simulink model "foc5"  (R2018a)
settings: Solver=ode45  StartTime=0.0  StopTime=0.5  MaxStep=2.0E-6  RelTol=1e-3
libraries: simulink x6, powerlib x4, powerlib_meascontrol x2
settings Model: Creator=R-YDL  LastModifiedBy=R-YDL

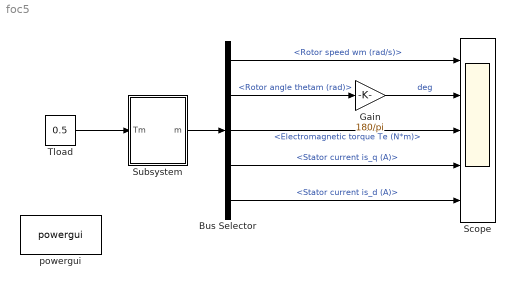
== system foc5 ==
  Bus Selector : BusSelector  OutputSignals=Rotor speed wm (rad/s),Rotor angle thetam (rad),Electromagnetic torque Te (N*m),Stator current is_q (A),Stator current is_d (A)
  Gain : Gain  Gain=180/pi
  Scope : Scope  NumInputPorts=5
  Subsystem : Subsystem  mask{Va=0, Vb=0, Vc=0, t0=0}
  Tload : Constant  Value=0.5
  powergui : powerlib/powergui  Priority=1  SimulationMode=Discrete  SampleTime=2e-6  frequency=60  Iterations=50  frequencyindice=0  Pbase=100e6  ErrMax=1e-4  UnitsV=kV  UnitsW=MW  buscounter=0  FunctionMessages=off  echomessages=off  EnableUseOfTLC=off  CurrentSourceSwitches=off  DisableSnubberDevices=off  DisableRonSwitches=off  DisableVfSwitches=off  DisplayEquations=off  SolverType=Tustin/Backward Euler (TBE)  Interpol=off  ExternalGateDelay=off  methode=off  Ts=100  x0status=blocks  SPID=on  SwTol=0  HookPort=off  RestoreLinks=warning  ResistiveCurrentMeasurement=off  Frange=[0:2:500]  Ylog=off  Xlog=on  ShowGrid=off  save=off  variable=ZData  structure=0  ZoomFFT=off  StartTime=0.0  cycles=1  DisplayStyle=1  fundamental=60  FreqAxis=off  MaxFrequency=1000  frequencyindicesteady=1  RmsSteady=1  display=off
  wires:
  Bus Selector/5 -> Scope/5  "<Stator current is_d (A)>"
  Bus Selector/4 -> Scope/4  "<Stator current is_q (A)>"
  Subsystem/1(m) -> Bus Selector/1
  Bus Selector/2 -> Gain/1  "<Rotor angle thetam (rad)>"
  Bus Selector/3 -> Scope/3  "<Electromagnetic torque Te (N*m)>"
  Gain/1 -> Scope/2  "deg"
  Bus Selector/1 -> Scope/1  "<Rotor speed wm (rad/s)>"
  Tload/1 -> Subsystem/1(Tm)

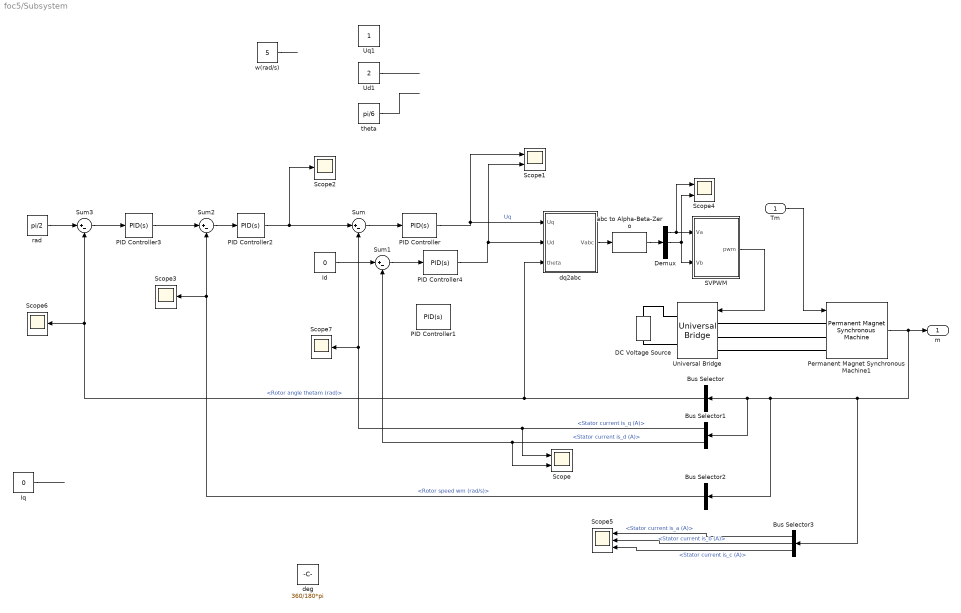
== system foc5/Subsystem ==
  Tm : Inport
  Bus Selector : BusSelector  OutputSignals=Rotor angle thetam (rad)
  Bus Selector1 : BusSelector  OutputSignals=Stator current is_q (A),Stator current is_d (A)
  Bus Selector2 : BusSelector  OutputSignals=Rotor speed wm (rad/s)
  Bus Selector3 : BusSelector  OutputSignals=Stator current is_a (A),Stator current is_b (A),Stator current is_c (A)
  DC Voltage Source : powerlib/Electrical Sources/DC Voltage Source  Amplitude=100  Measurements=None
  Demux : Demux  Outputs=3
  Id : Constant  Value=0
  Iq : Constant  Value=0
  PID Controller : simulink/Continuous/PID Controller  Controller=PID  TimeDomain=Continuous-time  SampleTime=-1  IntegratorMethod=Forward Euler  FilterMethod=Forward Euler  Form=Parallel  UseFilter=on  ControllerParametersSource=internal  P=50  I=5000  D=0  N=100  InitialConditionSource=internal  InitialConditionForIntegrator=0  InitialConditionForFilter=0  ExternalReset=none  LimitOutput=on  UpperSaturationLimit=100  LowerSaturationLimit=-100  LinearizeAsGain=on  AntiWindupMode=none  Kb=1  TrackingMode=off  Kt=1  PParamMin=[]  PParamMax=[]  IParamMin=[]  IParamMax=[]  DParamMin=[]  DParamMax=[]  NParamMin=[]  NParamMax=[]  KbParamMin=[]  KbParamMax=[]  KtParamMin=[]  KtParamMax=[]  POutMin=[]  POutMax=[]  IOutMin=[]  IOutMax=[]  DOutMin=[]  DOutMax=[]  NOutMin=[]  NOutMax=[]  KbOutMin=[]  KbOutMax=[]  KtOutMin=[]  KtOutMax=[]  IntegratorOutMin=[]  IntegratorOutMax=[]  FilterOutMin=[]  FilterOutMax=[]  SumOutMin=[]  SumOutMax=[]  SumI1OutMin=[]  SumI1OutMax=[]  SumI2OutMin=[]  SumI2OutMax=[]  SumI3OutMin=[]  SumI3OutMax=[]  SumDOutMin=[]  SumDOutMax=[]  SaturationOutMin=[]  SaturationOutMax=[]  IntegratorContinuousStateAttributes=''  IntegratorStateMustResolveToSignalObject=off  IntegratorRTWStateStorageClass=Auto  FilterContinuousStateAttributes=''  FilterStateMustResolveToSignalObject=off  FilterRTWStateStorageClass=Auto  DifferentiatorICPrevScaledInput=0  DifferentiatorOutMin=[]  DifferentiatorOutMax=[]  FilterDiffOutCoefMin=[]  FilterDiffOutCoefMax=[]  SumDenOutMin=[]  SumDenOutMax=[]  SumNumOutMin=[]  SumNumOutMax=[]  ReciprocalOutMin=[]  ReciprocalOutMax=[]  DivideOutMin=[]  DivideOutMax=[]  TunerSelectOption=Transfer Function Based (PID Tuner App)
  PID Controller1 : simulink/Continuous/PID Controller  Controller=PID  TimeDomain=Continuous-time  SampleTime=-1  IntegratorMethod=Forward Euler  FilterMethod=Forward Euler  Form=Parallel  UseFilter=on  ControllerParametersSource=internal  P=50  I=5000  D=0  N=100  InitialConditionSource=internal  InitialConditionForIntegrator=0  InitialConditionForFilter=0  ExternalReset=none  LimitOutput=on  UpperSaturationLimit=100  LowerSaturationLimit=-100  LinearizeAsGain=on  AntiWindupMode=none  Kb=1  TrackingMode=off  Kt=1  PParamMin=[]  PParamMax=[]  IParamMin=[]  IParamMax=[]  DParamMin=[]  DParamMax=[]  NParamMin=[]  NParamMax=[]  KbParamMin=[]  KbParamMax=[]  KtParamMin=[]  KtParamMax=[]  POutMin=[]  POutMax=[]  IOutMin=[]  IOutMax=[]  DOutMin=[]  DOutMax=[]  NOutMin=[]  NOutMax=[]  KbOutMin=[]  KbOutMax=[]  KtOutMin=[]  KtOutMax=[]  IntegratorOutMin=[]  IntegratorOutMax=[]  FilterOutMin=[]  FilterOutMax=[]  SumOutMin=[]  SumOutMax=[]  SumI1OutMin=[]  SumI1OutMax=[]  SumI2OutMin=[]  SumI2OutMax=[]  SumI3OutMin=[]  SumI3OutMax=[]  SumDOutMin=[]  SumDOutMax=[]  SaturationOutMin=[]  SaturationOutMax=[]  IntegratorContinuousStateAttributes=''  IntegratorStateMustResolveToSignalObject=off  IntegratorRTWStateStorageClass=Auto  FilterContinuousStateAttributes=''  FilterStateMustResolveToSignalObject=off  FilterRTWStateStorageClass=Auto  DifferentiatorICPrevScaledInput=0  DifferentiatorOutMin=[]  DifferentiatorOutMax=[]  FilterDiffOutCoefMin=[]  FilterDiffOutCoefMax=[]  SumDenOutMin=[]  SumDenOutMax=[]  SumNumOutMin=[]  SumNumOutMax=[]  ReciprocalOutMin=[]  ReciprocalOutMax=[]  DivideOutMin=[]  DivideOutMax=[]  TunerSelectOption=Transfer Function Based (PID Tuner App)
  PID Controller2 : simulink/Continuous/PID Controller  Controller=PID  TimeDomain=Continuous-time  SampleTime=-1  IntegratorMethod=Forward Euler  FilterMethod=Forward Euler  Form=Parallel  UseFilter=on  ControllerParametersSource=internal  P=20  I=500  D=0  N=100  InitialConditionSource=internal  InitialConditionForIntegrator=0  InitialConditionForFilter=0  ExternalReset=none  LimitOutput=on  UpperSaturationLimit=100  LowerSaturationLimit=-100  LinearizeAsGain=on  AntiWindupMode=none  Kb=1  TrackingMode=off  Kt=1  PParamMin=[]  PParamMax=[]  IParamMin=[]  IParamMax=[]  DParamMin=[]  DParamMax=[]  NParamMin=[]  NParamMax=[]  KbParamMin=[]  KbParamMax=[]  KtParamMin=[]  KtParamMax=[]  POutMin=[]  POutMax=[]  IOutMin=[]  IOutMax=[]  DOutMin=[]  DOutMax=[]  NOutMin=[]  NOutMax=[]  KbOutMin=[]  KbOutMax=[]  KtOutMin=[]  KtOutMax=[]  IntegratorOutMin=[]  IntegratorOutMax=[]  FilterOutMin=[]  FilterOutMax=[]  SumOutMin=[]  SumOutMax=[]  SumI1OutMin=[]  SumI1OutMax=[]  SumI2OutMin=[]  SumI2OutMax=[]  SumI3OutMin=[]  SumI3OutMax=[]  SumDOutMin=[]  SumDOutMax=[]  SaturationOutMin=[]  SaturationOutMax=[]  IntegratorContinuousStateAttributes=''  IntegratorStateMustResolveToSignalObject=off  IntegratorRTWStateStorageClass=Auto  FilterContinuousStateAttributes=''  FilterStateMustResolveToSignalObject=off  FilterRTWStateStorageClass=Auto  DifferentiatorICPrevScaledInput=0  DifferentiatorOutMin=[]  DifferentiatorOutMax=[]  FilterDiffOutCoefMin=[]  FilterDiffOutCoefMax=[]  SumDenOutMin=[]  SumDenOutMax=[]  SumNumOutMin=[]  SumNumOutMax=[]  ReciprocalOutMin=[]  ReciprocalOutMax=[]  DivideOutMin=[]  DivideOutMax=[]  TunerSelectOption=Transfer Function Based (PID Tuner App)
  PID Controller3 : simulink/Continuous/PID Controller  Controller=PID  TimeDomain=Continuous-time  SampleTime=-1  IntegratorMethod=Forward Euler  FilterMethod=Forward Euler  Form=Parallel  UseFilter=on  ControllerParametersSource=internal  P=3  I=0  D=0  N=100  InitialConditionSource=internal  InitialConditionForIntegrator=0  InitialConditionForFilter=0  ExternalReset=none  LimitOutput=on  UpperSaturationLimit=100  LowerSaturationLimit=-100  LinearizeAsGain=on  AntiWindupMode=none  Kb=1  TrackingMode=off  Kt=1  PParamMin=[]  PParamMax=[]  IParamMin=[]  IParamMax=[]  DParamMin=[]  DParamMax=[]  NParamMin=[]  NParamMax=[]  KbParamMin=[]  KbParamMax=[]  KtParamMin=[]  KtParamMax=[]  POutMin=[]  POutMax=[]  IOutMin=[]  IOutMax=[]  DOutMin=[]  DOutMax=[]  NOutMin=[]  NOutMax=[]  KbOutMin=[]  KbOutMax=[]  KtOutMin=[]  KtOutMax=[]  IntegratorOutMin=[]  IntegratorOutMax=[]  FilterOutMin=[]  FilterOutMax=[]  SumOutMin=[]  SumOutMax=[]  SumI1OutMin=[]  SumI1OutMax=[]  SumI2OutMin=[]  SumI2OutMax=[]  SumI3OutMin=[]  SumI3OutMax=[]  SumDOutMin=[]  SumDOutMax=[]  SaturationOutMin=[]  SaturationOutMax=[]  IntegratorContinuousStateAttributes=''  IntegratorStateMustResolveToSignalObject=off  IntegratorRTWStateStorageClass=Auto  FilterContinuousStateAttributes=''  FilterStateMustResolveToSignalObject=off  FilterRTWStateStorageClass=Auto  DifferentiatorICPrevScaledInput=0  DifferentiatorOutMin=[]  DifferentiatorOutMax=[]  FilterDiffOutCoefMin=[]  FilterDiffOutCoefMax=[]  SumDenOutMin=[]  SumDenOutMax=[]  SumNumOutMin=[]  SumNumOutMax=[]  ReciprocalOutMin=[]  ReciprocalOutMax=[]  DivideOutMin=[]  DivideOutMax=[]  TunerSelectOption=Transfer Function Based (PID Tuner App)
  PID Controller4 : simulink/Continuous/PID Controller  Controller=PID  TimeDomain=Continuous-time  SampleTime=-1  IntegratorMethod=Forward Euler  FilterMethod=Forward Euler  Form=Parallel  UseFilter=on  ControllerParametersSource=internal  P=50  I=5000  D=0  N=100  InitialConditionSource=internal  InitialConditionForIntegrator=0  InitialConditionForFilter=0  ExternalReset=none  LimitOutput=on  UpperSaturationLimit=100  LowerSaturationLimit=-100  LinearizeAsGain=on  AntiWindupMode=none  Kb=1  TrackingMode=off  Kt=1  PParamMin=[]  PParamMax=[]  IParamMin=[]  IParamMax=[]  DParamMin=[]  DParamMax=[]  NParamMin=[]  NParamMax=[]  KbParamMin=[]  KbParamMax=[]  KtParamMin=[]  KtParamMax=[]  POutMin=[]  POutMax=[]  IOutMin=[]  IOutMax=[]  DOutMin=[]  DOutMax=[]  NOutMin=[]  NOutMax=[]  KbOutMin=[]  KbOutMax=[]  KtOutMin=[]  KtOutMax=[]  IntegratorOutMin=[]  IntegratorOutMax=[]  FilterOutMin=[]  FilterOutMax=[]  SumOutMin=[]  SumOutMax=[]  SumI1OutMin=[]  SumI1OutMax=[]  SumI2OutMin=[]  SumI2OutMax=[]  SumI3OutMin=[]  SumI3OutMax=[]  SumDOutMin=[]  SumDOutMax=[]  SaturationOutMin=[]  SaturationOutMax=[]  IntegratorContinuousStateAttributes=''  IntegratorStateMustResolveToSignalObject=off  IntegratorRTWStateStorageClass=Auto  FilterContinuousStateAttributes=''  FilterStateMustResolveToSignalObject=off  FilterRTWStateStorageClass=Auto  DifferentiatorICPrevScaledInput=0  DifferentiatorOutMin=[]  DifferentiatorOutMax=[]  FilterDiffOutCoefMin=[]  FilterDiffOutCoefMax=[]  SumDenOutMin=[]  SumDenOutMax=[]  SumNumOutMin=[]  SumNumOutMax=[]  ReciprocalOutMin=[]  ReciprocalOutMax=[]  DivideOutMin=[]  DivideOutMax=[]  TunerSelectOption=Transfer Function Based (PID Tuner App)
  Permanent Magnet Synchronous Machine1 : powerlib/Machines/Permanent Magnet Synchronous Machine  NbPhases=3  FluxDistribution=Sinusoidal  RotorType=Round  MechanicalLoad=Torque Tm  PresetModel=No  ShowDetailedParameters=on  MeasurementBus=off  Resistance=7  Inductance=8.5e-3  dqInductances=[8.5e-3,8.5e-3]  La=0.000395  MachineConstant=Flux linkage established by magnets (V.s)  Flux=0.1194  VoltageCst=21.6568  TorqueCst=0.1791  Flat=120  Mechanical=[0.0027 0.0424924 1 0]  PolePairs=4  InitialConditions=[0,t0, 0,0]  InitialConditions5ph=[0 0 0 0 0 0]  TsPowergui=0  TsBlock=-1  RefAngle=Aligned with phase A axis (original Park)
      settings: SourceProductName=Simscape Power Systems
  SVPWM : Subsystem  mask{T=1e-4, Ts=2e-6, Td=2e-6, Vdc=12}
      mask prompts: T "载波周期T(s)"; Ts "采样周期Ts"; Td "死区时间Td"; Vdc "直流母线电压Vdc"
  Scope : Scope  NumInputPorts=2
  Scope1 : Scope  NumInputPorts=2
  Scope{2..3,6..7} (4 alike) : Scope
  Scope4 : Scope  NumInputPorts=2
  Scope5 : Scope  NumInputPorts=3
  Sum{,1..3} (4 alike) : Sum  Inputs=|+-
  Ud1 : Constant  Value=2
  Universal Bridge : powerlib/Power Electronics/Universal Bridge  Arms=3  SnubberResistance=1e5  SnubberCapacitance=inf  Device=IGBT / Diodes  Ron=1e-3  Lon=0  ForwardVoltages="[  0  0  ]"  ForwardVoltage=0  GTOparameters=[ 10e-6 , 20e-6 ]  IGBTparameters=[ 1e-6 , 2e-6 ]  Measurements=None  Measurements_2=None  converterType=Rectifier
  Uq1 : Constant
  abc to Alpha-Beta-Zero : powerlib_meascontrol/Transformations/abc to Alpha-Beta-Zero
      settings: SourceProductName=Simscape Power Systems
  deg : Constant  Value=360/180*pi
  dq2abc : Subsystem
  rad : Constant  Value=pi/2
  theta : Constant  Value=pi/6
  w(rad/s) : Constant  Value=5
  m : Outport
  wires:
  Tm/1 -> Permanent Magnet Synchronous Machine1/1
  Permanent Magnet Synchronous Machine1/1 -> m/1, Bus Selector3/1, Bus Selector2/1, Bus Selector1/1, Bus Selector/1
  Sum/1 -> PID Controller/1
  Id/1 -> Sum1/1
  PID Controller/1 -> dq2abc/1(Uq), Scope1/1  "Uq"
  Bus Selector1/1 -> Scope/1, Scope7/1, Sum/2  "<Stator current is_q (A)>"
  Bus Selector1/2 -> Scope/2, Sum1/2  "<Stator current is_d (A)>"
  PID Controller2/1 -> Sum/1, Scope2/1
  Sum2/1 -> PID Controller2/1
  Bus Selector2/1 -> Scope3/1, Sum2/2  "<Rotor speed wm (rad/s)>"
  SVPWM/1(pwm) -> Universal Bridge/1
  Demux/1 -> Scope4/1, SVPWM/1(Va)
  Demux/2 -> Scope4/2, SVPWM/2(Vb)
  dq2abc/1(Vabc) -> abc to Alpha-Beta-Zero/1
  abc to Alpha-Beta-Zero/1 -> Demux/1
  Bus Selector3/1 -> Scope5/1  "<Stator current is_a (A)>"
  Bus Selector3/2 -> Scope5/2  "<Stator current is_b (A)>"
  Bus Selector3/3 -> Scope5/3  "<Stator current is_c (A)>"
  Bus Selector/1 -> dq2abc/3(theta), Scope6/1, Sum3/2  "<Rotor angle thetam (rad)>"
  rad/1 -> Sum3/1
  Sum3/1 -> PID Controller3/1
  w(rad/s)/1 -> ?
  PID Controller3/1 -> Sum2/1
  theta/1 -> ?
  Ud1/1 -> ?
  PID Controller4/1 -> Scope1/2, dq2abc/2(Ud)
  Sum1/1 -> PID Controller4/1
  Iq/1 -> ?
  connections:
  Universal Bridge/LConn2 -- Permanent Magnet Synchronous Machine1/LConn2
  Universal Bridge/LConn1 -- Permanent Magnet Synchronous Machine1/LConn1
  Universal Bridge/LConn3 -- Permanent Magnet Synchronous Machine1/LConn3
  Universal Bridge/RConn1 -- DC Voltage Source/RConn1
  Universal Bridge/RConn2 -- DC Voltage Source/LConn1

== system foc5/Subsystem/SVPWM ==
  Va : Inport
  Vb : Inport  Port=2
  Constant : Constant  Value=2/3*Vdc
  Divide : Product  Inputs=*/
  Divide1 : Product  Inputs=*/
  PWM : Subsystem
  Scope1 : Scope
  Scope2 : Scope
  Sec : Subsystem
  Subsystem5 : Subsystem
  pwm : Outport
  wires:
  Subsystem5/1(m(a,b,c)) -> Scope1/1, PWM/1("m_(a,b,c) ")
  PWM/1(pwm) -> pwm/1
  Sec/1(sec) -> Subsystem5/1(sec), Scope2/1
  Va/1 -> Divide/1
  Divide/1 -> Subsystem5/2(Va), Sec/1(Va)
  Vb/1 -> Divide1/1
  Divide1/1 -> Sec/2(Vb), Subsystem5/3(Vb)
  Constant/1 -> Divide1/2, Divide/2

== system foc5/Subsystem/dq2abc ==
  Uq : Inport
  Ud : Inport  Port=2
  theta : Inport  Port=3
  Mux : Mux  Inputs=3
  Subsystem : Subsystem
  Subsystem1 : Subsystem
  Subsystem3 : Subsystem
  Vabc : Outport
  wires:
  theta/1 -> Subsystem/3(theta), Subsystem1/3(theta), Subsystem3/3(theta)
  Ud/1 -> Subsystem3/2(Ud), Subsystem1/2(Ud), Subsystem/2(Ud)
  Uq/1 -> Subsystem3/1(Uq), Subsystem1/1(Uq), Subsystem/1(Uq)
  Subsystem/1(V) -> Mux/1
  Subsystem1/1(V) -> Mux/2
  Subsystem3/1(V) -> Mux/3
  Mux/1 -> Vabc/1

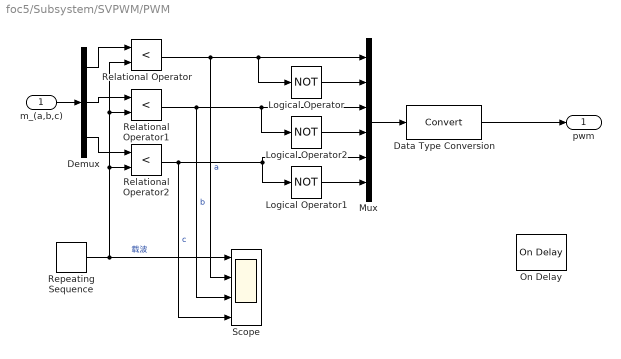
== system foc5/Subsystem/SVPWM/PWM ==
  "m_(a,b,c) " : Inport
  Data Type Conversion : DataTypeConversion
  Demux : Demux  Outputs=3
  Logical Operator : Logic  Operator=NOT  AllPortsSameDT=off  OutDataTypeStr=boolean
  Logical Operator1 : Logic  Operator=NOT  AllPortsSameDT=off  OutDataTypeStr=boolean
  Logical Operator2 : Logic  Operator=NOT  AllPortsSameDT=off  OutDataTypeStr=boolean
  Mux : Mux  Inputs=6
  On Delay : powerlib_meascontrol/Logic/On Delay  DelayType=On delay  delay=Td  ic=0  Ts=Ts
      settings: SourceProductName=Simscape Power Systems
  Relational Operator : RelationalOperator  Operator=<  OutDataTypeStr=boolean  RndMeth=Simplest
  Relational Operator1 : RelationalOperator  Operator=<  OutDataTypeStr=boolean  RndMeth=Simplest
  Relational Operator2 : RelationalOperator  Operator=<  OutDataTypeStr=boolean  RndMeth=Simplest
  Repeating Sequence : simulink/Sources/Repeating Sequence  rep_seq_t=[0 0.5 1]*T  rep_seq_y=[0 0.5 0]*T
  Scope : Scope  NumInputPorts=4
  pwm : Outport
  wires:
  Repeating Sequence/1 -> Relational Operator/2, Relational Operator1/2, Relational Operator2/2, Scope/1  "载波"
  Relational Operator/1 -> Mux/1, Logical Operator/1, Scope/2  "a"
  Relational Operator1/1 -> Logical Operator2/1, Mux/3, Scope/3  "b"
  Relational Operator2/1 -> Logical Operator1/1, Mux/5, Scope/4  "c"
  "m_(a,b,c) "/1 -> Demux/1
  Demux/1 -> Relational Operator/1
  Demux/2 -> Relational Operator1/1
  Demux/3 -> Relational Operator2/1
  Logical Operator/1 -> Mux/2
  Logical Operator2/1 -> Mux/4
  Logical Operator1/1 -> Mux/6
  Mux/1 -> Data Type Conversion/1
  Data Type Conversion/1 -> pwm/1

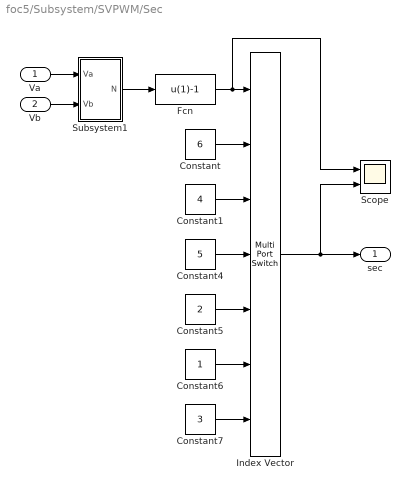
== system foc5/Subsystem/SVPWM/Sec ==
  Va : Inport
  Vb : Inport  Port=2
  Constant : Constant  Value=6
  Constant1 : Constant  Value=4
  Constant4 : Constant  Value=5
  Constant5 : Constant  Value=2
  Constant6 : Constant
  Constant7 : Constant  Value=3
  Fcn : Fcn  Expr=u(1)-1
  Index Vector : MultiPortSwitch  DataPortOrder=Zero-based contiguous  Inputs=6  zeroidx=on
  Scope : Scope  NumInputPorts=2
  Subsystem1 : Subsystem
  sec : Outport
  wires:
  Constant4/1 -> Index Vector/4
  Constant7/1 -> Index Vector/7
  Constant6/1 -> Index Vector/6
  Constant5/1 -> Index Vector/5
  Constant1/1 -> Index Vector/3
  Subsystem1/1("N ") -> Fcn/1
  Fcn/1 -> Scope/1, Index Vector/1
  Constant/1 -> Index Vector/2
  Va/1 -> Subsystem1/1(Va)
  Vb/1 -> Subsystem1/2("Vb ")
  Index Vector/1 -> sec/1, Scope/2

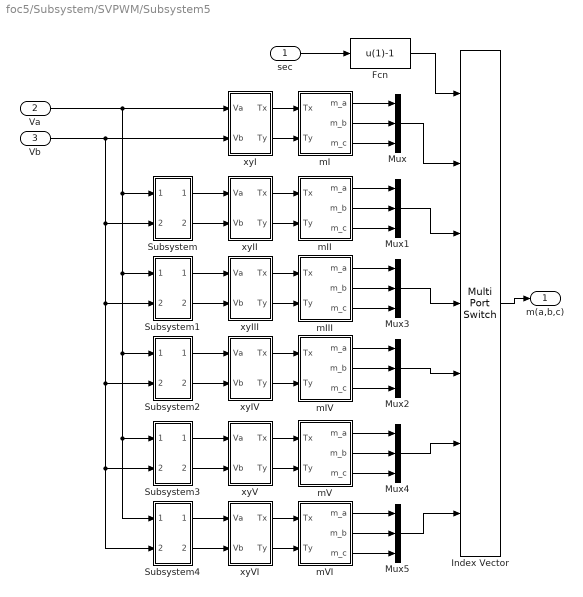
== system foc5/Subsystem/SVPWM/Subsystem5 ==
  sec : Inport
  Va : Inport  Port=2
  Vb : Inport  Port=3
  Fcn : Fcn  Expr=u(1)-1
  Index Vector : MultiPortSwitch  DataPortOrder=Zero-based contiguous  Inputs=6  zeroidx=on
  Mux{,1..5} (6 alike) : Mux  Inputs=3
  Subsystem : Subsystem
  Subsystem1 : Subsystem
  Subsystem2 : Subsystem
  Subsystem3 : Subsystem
  Subsystem4 : Subsystem
  mI : Subsystem
  mII : Subsystem
  mIII : Subsystem
  mIV : Subsystem
  mV : Subsystem
  mVI : Subsystem
  xyI : Subsystem
  xyII : Subsystem
  xyIII : Subsystem
  xyIV : Subsystem
  xyV : Subsystem
  xyVI : Subsystem
  m(a,b,c) : Outport
  wires:
  Subsystem2/1(Va') -> xyIV/1(Va)
  xyVI/2(Ty) -> mVI/2(Ty)
  mVI/1(m_a) -> Mux5/1
  Vb/1 -> Subsystem2/2(Vb), Subsystem4/2(Vb), Subsystem3/2(Vb), Subsystem1/2(Vb), Subsystem/2(Vb), xyI/2("Vb ")
  Subsystem2/2(Vb') -> xyIV/2("Vb ")
  mIV/3(m_c) -> Mux2/3
  Subsystem/1(Va') -> xyII/1(Va)
  Mux1/1 -> Index Vector/3
  Subsystem1/2(Vb') -> xyIII/2("Vb ")
  Va/1 -> Subsystem/1(Va), Subsystem4/1(Va), Subsystem3/1(Va), Subsystem2/1(Va), Subsystem1/1(Va), xyI/1(Va)
  mVI/2(m_b) -> Mux5/2
  Subsystem3/1(Va') -> xyV/1(Va)
  Mux/1 -> Index Vector/2
  xyIV/2(Ty) -> mIV/2(Ty)
  Mux4/1 -> Index Vector/6
  mVI/3(m_c) -> Mux5/3
  xyIV/1(Tx) -> mIV/1(Tx)
  xyI/1(Tx) -> mI/1("Tx ")
  mIV/2(m_b) -> Mux2/2
  Mux3/1 -> Index Vector/4
  xyI/2(Ty) -> mI/2("Ty ")
  Subsystem1/1(Va') -> xyIII/1(Va)
  mI/3(m_c) -> Mux/3
  xyIII/2(Ty) -> mIII/2(Ty)
  mI/2(m_b) -> Mux/2
  mI/1(m_a) -> Mux/1
  Subsystem4/1(Va') -> xyVI/1(Va)
  mIV/1(m_a) -> Mux2/1
  xyIII/1(Tx) -> mIII/1(Tx)
  xyII/2(Ty) -> mII/2("Ty ")
  xyII/1(Tx) -> mII/1("Tx ")
  Subsystem3/2(Vb') -> xyV/2("Vb ")
  Mux2/1 -> Index Vector/5
  Subsystem4/2(Vb') -> xyVI/2("Vb ")
  Mux5/1 -> Index Vector/7
  Subsystem/2(Vb') -> xyII/2("Vb ")
  xyVI/1(Tx) -> mVI/1(Tx)
  sec/1 -> Fcn/1
  Fcn/1 -> Index Vector/1
  mII/1(m_a) -> Mux1/1
  mII/2(m_b) -> Mux1/2
  mII/3(m_c) -> Mux1/3
  mIII/1(m_a) -> Mux3/1
  mIII/2(m_b) -> Mux3/2
  mIII/3(m_c) -> Mux3/3
  mV/1(m_a) -> Mux4/1
  mV/2(m_b) -> Mux4/2
  mV/3(m_c) -> Mux4/3
  Index Vector/1 -> m(a,b,c)/1
  xyV/1(Tx) -> mV/1(Tx)
  xyV/2(Ty) -> mV/2(Ty)

== system foc5/Subsystem/dq2abc/Subsystem ==
  Uq : Inport
  Ud : Inport  Port=2
  theta : Inport  Port=3
  Constant : Constant  Value=0
  Product : Product
  Product1 : Product
  Sum : Sum  Inputs=|-+
  Sum1 : Sum  Inputs=|++
  Trigonometric Function : Trigonometry
  Trigonometric Function1 : Trigonometry  Operator=cos
  V : Outport
  wires:
  Uq/1 -> Product/1
  Trigonometric Function1/1 -> Product1/2
  Trigonometric Function/1 -> Product/2
  Product1/1 -> Sum/2
  Product/1 -> Sum/1
  Sum/1 -> V/1
  Ud/1 -> Product1/1
  Sum1/1 -> Trigonometric Function/1, Trigonometric Function1/1
  theta/1 -> Sum1/1
  Constant/1 -> Sum1/2

== system foc5/Subsystem/dq2abc/Subsystem1 ==
  Uq : Inport
  Ud : Inport  Port=2
  theta : Inport  Port=3
  Constant : Constant  Value=-2*pi/3
  Product : Product
  Product1 : Product
  Sum : Sum  Inputs=|-+
  Sum1 : Sum  Inputs=|++
  Trigonometric Function : Trigonometry
  Trigonometric Function1 : Trigonometry  Operator=cos
  V : Outport
  wires:
  Uq/1 -> Product/1
  Trigonometric Function1/1 -> Product1/2
  Trigonometric Function/1 -> Product/2
  Product1/1 -> Sum/2
  Product/1 -> Sum/1
  Sum/1 -> V/1
  Ud/1 -> Product1/1
  Sum1/1 -> Trigonometric Function/1, Trigonometric Function1/1
  theta/1 -> Sum1/1
  Constant/1 -> Sum1/2

== system foc5/Subsystem/dq2abc/Subsystem3 ==
  Uq : Inport
  Ud : Inport  Port=2
  theta : Inport  Port=3
  Constant : Constant  Value=2*pi/3
  Product : Product
  Product1 : Product
  Sum : Sum  Inputs=|-+
  Sum1 : Sum  Inputs=|++
  Trigonometric Function : Trigonometry
  Trigonometric Function1 : Trigonometry  Operator=cos
  V : Outport
  wires:
  Uq/1 -> Product/1
  Trigonometric Function1/1 -> Product1/2
  Trigonometric Function/1 -> Product/2
  Product1/1 -> Sum/2
  Product/1 -> Sum/1
  Sum/1 -> V/1
  Ud/1 -> Product1/1
  Sum1/1 -> Trigonometric Function/1, Trigonometric Function1/1
  theta/1 -> Sum1/1
  Constant/1 -> Sum1/2

== system foc5/Subsystem/SVPWM/Sec/Subsystem1 ==
  Va : Inport
  "Vb " : Inport  Port=2
  Gain : Gain
  Gain1 : Gain  Gain=2
  Gain2 : Gain  Gain=4
  Scope : Scope  NumInputPorts=4
  Subsystem : Subsystem
  Subsystem1 : Subsystem
  Subsystem2 : Subsystem
  Sum : Sum  Inputs=+++
  "N " : Outport
  wires:
  Va/1 -> Subsystem/1(Va), Subsystem1/1(Va)
  Subsystem2/1(C) -> Gain2/1
  Subsystem1/1(B) -> Gain1/1
  Subsystem/1(A) -> Gain/1
  "Vb "/1 -> Subsystem2/1("Vb "), Subsystem1/2("Vb "), Subsystem/2("Vb ")
  Gain/1 -> Scope/1, Sum/1
  Gain1/1 -> Sum/2, Scope/2
  Gain2/1 -> Scope/3, Sum/3
  Sum/1 -> "N "/1, Scope/4  "N=1*A+2*B+4*C"

== system foc5/Subsystem/SVPWM/Subsystem5/Subsystem ==
  Va : Inport
  Vb : Inport  Port=2
  Add : Sum  Inputs=+-
  Complex to Magnitude-Angle : ComplexToMagnitudeAngle
  Complex to Real-Imag : ComplexToRealImag
  Constant : Constant
  Gain : Gain  Gain=pi/3
  Magnitude-Angle to Complex : MagnitudeAngleToComplex
  Real-Imag to Complex : RealImagToComplex
  Va' : Outport
  Vb' : Outport  Port=2
  wires:
  Complex to Magnitude-Angle/2 -> Add/1
  Gain/1 -> Add/2
  Complex to Real-Imag/1 -> Va'/1
  Complex to Real-Imag/2 -> Vb'/1
  Complex to Magnitude-Angle/1 -> Magnitude-Angle to Complex/1
  Va/1 -> Real-Imag to Complex/1
  Vb/1 -> Real-Imag to Complex/2
  Real-Imag to Complex/1 -> Complex to Magnitude-Angle/1
  Add/1 -> Magnitude-Angle to Complex/2
  Magnitude-Angle to Complex/1 -> Complex to Real-Imag/1
  Constant/1 -> Gain/1

== system foc5/Subsystem/SVPWM/Subsystem5/Subsystem1 ==
  Va : Inport
  Vb : Inport  Port=2
  Add : Sum  Inputs=+-
  Complex to Magnitude-Angle : ComplexToMagnitudeAngle
  Complex to Real-Imag : ComplexToRealImag
  Constant : Constant  Value=2
  Gain : Gain  Gain=pi/3
  Magnitude-Angle to Complex : MagnitudeAngleToComplex
  Real-Imag to Complex : RealImagToComplex
  Va' : Outport
  Vb' : Outport  Port=2
  wires:
  Complex to Magnitude-Angle/2 -> Add/1
  Gain/1 -> Add/2
  Complex to Real-Imag/1 -> Va'/1
  Complex to Real-Imag/2 -> Vb'/1
  Complex to Magnitude-Angle/1 -> Magnitude-Angle to Complex/1
  Va/1 -> Real-Imag to Complex/1
  Vb/1 -> Real-Imag to Complex/2
  Real-Imag to Complex/1 -> Complex to Magnitude-Angle/1
  Add/1 -> Magnitude-Angle to Complex/2
  Magnitude-Angle to Complex/1 -> Complex to Real-Imag/1
  Constant/1 -> Gain/1

== system foc5/Subsystem/SVPWM/Subsystem5/Subsystem2 ==
  Va : Inport
  Vb : Inport  Port=2
  Add : Sum  Inputs=+-
  Complex to Magnitude-Angle : ComplexToMagnitudeAngle
  Complex to Real-Imag : ComplexToRealImag
  Constant : Constant  Value=3
  Gain : Gain  Gain=pi/3
  Magnitude-Angle to Complex : MagnitudeAngleToComplex
  Real-Imag to Complex : RealImagToComplex
  Va' : Outport
  Vb' : Outport  Port=2
  wires:
  Complex to Magnitude-Angle/2 -> Add/1
  Gain/1 -> Add/2
  Complex to Real-Imag/1 -> Va'/1
  Complex to Real-Imag/2 -> Vb'/1
  Complex to Magnitude-Angle/1 -> Magnitude-Angle to Complex/1
  Va/1 -> Real-Imag to Complex/1
  Vb/1 -> Real-Imag to Complex/2
  Real-Imag to Complex/1 -> Complex to Magnitude-Angle/1
  Add/1 -> Magnitude-Angle to Complex/2
  Magnitude-Angle to Complex/1 -> Complex to Real-Imag/1
  Constant/1 -> Gain/1

== system foc5/Subsystem/SVPWM/Subsystem5/Subsystem3 ==
  Va : Inport
  Vb : Inport  Port=2
  Add : Sum  Inputs=+-
  Complex to Magnitude-Angle : ComplexToMagnitudeAngle
  Complex to Real-Imag : ComplexToRealImag
  Constant : Constant  Value=4
  Gain : Gain  Gain=pi/3
  Magnitude-Angle to Complex : MagnitudeAngleToComplex
  Real-Imag to Complex : RealImagToComplex
  Va' : Outport
  Vb' : Outport  Port=2
  wires:
  Complex to Magnitude-Angle/2 -> Add/1
  Gain/1 -> Add/2
  Complex to Real-Imag/1 -> Va'/1
  Complex to Real-Imag/2 -> Vb'/1
  Complex to Magnitude-Angle/1 -> Magnitude-Angle to Complex/1
  Va/1 -> Real-Imag to Complex/1
  Vb/1 -> Real-Imag to Complex/2
  Real-Imag to Complex/1 -> Complex to Magnitude-Angle/1
  Add/1 -> Magnitude-Angle to Complex/2
  Magnitude-Angle to Complex/1 -> Complex to Real-Imag/1
  Constant/1 -> Gain/1

== system foc5/Subsystem/SVPWM/Subsystem5/Subsystem4 ==
  Va : Inport
  Vb : Inport  Port=2
  Add : Sum  Inputs=+-
  Complex to Magnitude-Angle : ComplexToMagnitudeAngle
  Complex to Real-Imag : ComplexToRealImag
  Constant : Constant  Value=5
  Gain : Gain  Gain=pi/3
  Magnitude-Angle to Complex : MagnitudeAngleToComplex
  Real-Imag to Complex : RealImagToComplex
  Va' : Outport
  Vb' : Outport  Port=2
  wires:
  Complex to Magnitude-Angle/2 -> Add/1
  Gain/1 -> Add/2
  Complex to Real-Imag/1 -> Va'/1
  Complex to Real-Imag/2 -> Vb'/1
  Complex to Magnitude-Angle/1 -> Magnitude-Angle to Complex/1
  Va/1 -> Real-Imag to Complex/1
  Vb/1 -> Real-Imag to Complex/2
  Real-Imag to Complex/1 -> Complex to Magnitude-Angle/1
  Add/1 -> Magnitude-Angle to Complex/2
  Magnitude-Angle to Complex/1 -> Complex to Real-Imag/1
  Constant/1 -> Gain/1

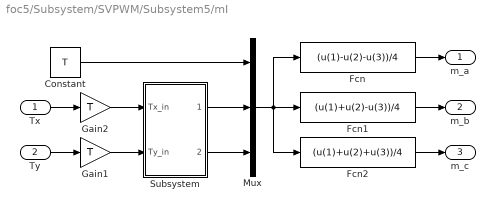
== system foc5/Subsystem/SVPWM/Subsystem5/mI ==
  "Tx " : Inport
  "Ty " : Inport  Port=2
  Constant : Constant  Value=T
  Fcn : Fcn  Expr=(u(1)-u(2)-u(3))/4
  Fcn1 : Fcn  Expr=(u(1)+u(2)-u(3))/4
  Fcn2 : Fcn  Expr=(u(1)+u(2)+u(3))/4
  Gain1 : Gain  Gain=T
  Gain2 : Gain  Gain=T
  Mux : Mux  Inputs=3
  Subsystem : Subsystem
  m_a : Outport
  m_b : Outport  Port=2
  m_c : Outport  Port=3
  wires:
  "Ty "/1 -> Gain1/1
  "Tx "/1 -> Gain2/1
  Gain1/1 -> Subsystem/2(Ty_in)
  Constant/1 -> Mux/1
  Fcn/1 -> m_a/1
  Fcn1/1 -> m_b/1
  Fcn2/1 -> m_c/1
  Mux/1 -> Fcn2/1, Fcn1/1, Fcn/1
  Gain2/1 -> Subsystem/1(Tx_in)
  Subsystem/2(Ty_out) -> Mux/3
  Subsystem/1(Tx_out) -> Mux/2

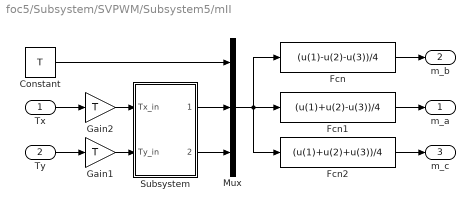
== system foc5/Subsystem/SVPWM/Subsystem5/mII ==
  "Tx " : Inport
  "Ty " : Inport  Port=2
  Constant : Constant  Value=T
  Fcn : Fcn  Expr=(u(1)-u(2)-u(3))/4
  Fcn1 : Fcn  Expr=(u(1)+u(2)-u(3))/4
  Fcn2 : Fcn  Expr=(u(1)+u(2)+u(3))/4
  Gain1 : Gain  Gain=T
  Gain2 : Gain  Gain=T
  Mux : Mux  Inputs=3
  Subsystem : Subsystem
  m_a : Outport
  m_b : Outport  Port=2
  m_c : Outport  Port=3
  wires:
  "Ty "/1 -> Gain1/1
  "Tx "/1 -> Gain2/1
  Constant/1 -> Mux/1
  Fcn2/1 -> m_c/1
  Mux/1 -> Fcn2/1, Fcn1/1, Fcn/1
  Fcn/1 -> m_b/1
  Fcn1/1 -> m_a/1
  Gain2/1 -> Subsystem/1(Tx_in)
  Gain1/1 -> Subsystem/2(Ty_in)
  Subsystem/1(Tx_out) -> Mux/2
  Subsystem/2(Ty_out) -> Mux/3

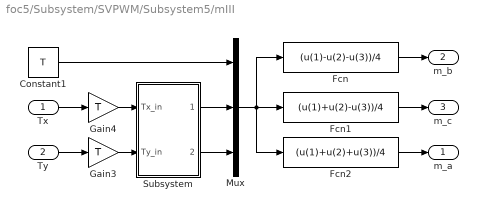
== system foc5/Subsystem/SVPWM/Subsystem5/mIII ==
  Tx : Inport
  Ty : Inport  Port=2
  Constant1 : Constant  Value=T
  Fcn : Fcn  Expr=(u(1)-u(2)-u(3))/4
  Fcn1 : Fcn  Expr=(u(1)+u(2)-u(3))/4
  Fcn2 : Fcn  Expr=(u(1)+u(2)+u(3))/4
  Gain3 : Gain  Gain=T
  Gain4 : Gain  Gain=T
  Mux : Mux  Inputs=3
  Subsystem : Subsystem
  m_a : Outport
  m_b : Outport  Port=2
  m_c : Outport  Port=3
  wires:
  Mux/1 -> Fcn2/1, Fcn1/1, Fcn/1
  Fcn/1 -> m_b/1
  Fcn1/1 -> m_c/1
  Fcn2/1 -> m_a/1
  Gain4/1 -> Subsystem/1(Tx_in)
  Gain3/1 -> Subsystem/2(Ty_in)
  Tx/1 -> Gain4/1
  Ty/1 -> Gain3/1
  Constant1/1 -> Mux/1
  Subsystem/1(Tx_out) -> Mux/2
  Subsystem/2(Ty_out) -> Mux/3

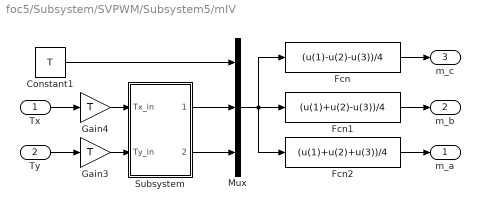
== system foc5/Subsystem/SVPWM/Subsystem5/mIV ==
  Tx : Inport
  Ty : Inport  Port=2
  Constant1 : Constant  Value=T
  Fcn : Fcn  Expr=(u(1)-u(2)-u(3))/4
  Fcn1 : Fcn  Expr=(u(1)+u(2)-u(3))/4
  Fcn2 : Fcn  Expr=(u(1)+u(2)+u(3))/4
  Gain3 : Gain  Gain=T
  Gain4 : Gain  Gain=T
  Mux : Mux  Inputs=3
  Subsystem : Subsystem
  m_a : Outport
  m_b : Outport  Port=2
  m_c : Outport  Port=3
  wires:
  Mux/1 -> Fcn2/1, Fcn1/1, Fcn/1
  Fcn2/1 -> m_a/1
  Fcn1/1 -> m_b/1
  Fcn/1 -> m_c/1
  Gain4/1 -> Subsystem/1(Tx_in)
  Gain3/1 -> Subsystem/2(Ty_in)
  Tx/1 -> Gain4/1
  Ty/1 -> Gain3/1
  Constant1/1 -> Mux/1
  Subsystem/1(Tx_out) -> Mux/2
  Subsystem/2(Ty_out) -> Mux/3

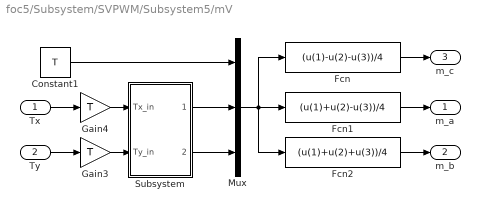
== system foc5/Subsystem/SVPWM/Subsystem5/mV ==
  Tx : Inport
  Ty : Inport  Port=2
  Constant1 : Constant  Value=T
  Fcn : Fcn  Expr=(u(1)-u(2)-u(3))/4
  Fcn1 : Fcn  Expr=(u(1)+u(2)-u(3))/4
  Fcn2 : Fcn  Expr=(u(1)+u(2)+u(3))/4
  Gain3 : Gain  Gain=T
  Gain4 : Gain  Gain=T
  Mux : Mux  Inputs=3
  Subsystem : Subsystem
  m_a : Outport
  m_b : Outport  Port=2
  m_c : Outport  Port=3
  wires:
  Mux/1 -> Fcn2/1, Fcn1/1, Fcn/1
  Fcn/1 -> m_c/1
  Fcn1/1 -> m_a/1
  Fcn2/1 -> m_b/1
  Gain4/1 -> Subsystem/1(Tx_in)
  Gain3/1 -> Subsystem/2(Ty_in)
  Ty/1 -> Gain3/1
  Tx/1 -> Gain4/1
  Constant1/1 -> Mux/1
  Subsystem/1(Tx_out) -> Mux/2
  Subsystem/2(Ty_out) -> Mux/3

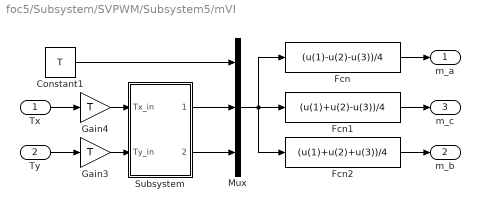
== system foc5/Subsystem/SVPWM/Subsystem5/mVI ==
  Tx : Inport
  Ty : Inport  Port=2
  Constant1 : Constant  Value=T
  Fcn : Fcn  Expr=(u(1)-u(2)-u(3))/4
  Fcn1 : Fcn  Expr=(u(1)+u(2)-u(3))/4
  Fcn2 : Fcn  Expr=(u(1)+u(2)+u(3))/4
  Gain3 : Gain  Gain=T
  Gain4 : Gain  Gain=T
  Mux : Mux  Inputs=3
  Subsystem : Subsystem
  m_a : Outport
  m_b : Outport  Port=2
  m_c : Outport  Port=3
  wires:
  Mux/1 -> Fcn2/1, Fcn1/1, Fcn/1
  Fcn2/1 -> m_b/1
  Fcn/1 -> m_a/1
  Fcn1/1 -> m_c/1
  Subsystem/1(Tx_out) -> Mux/2
  Constant1/1 -> Mux/1
  Gain4/1 -> Subsystem/1(Tx_in)
  Subsystem/2(Ty_out) -> Mux/3
  Ty/1 -> Gain3/1
  Gain3/1 -> Subsystem/2(Ty_in)
  Tx/1 -> Gain4/1

== system foc5/Subsystem/SVPWM/Subsystem5/xyI ==
  Va : Inport
  "Vb " : Inport  Port=2
  Gain : Gain  Gain=1/sqrt(3)
  Gain1 : Gain  Gain=2
  Sum : Sum  Inputs=|+-
  Tx : Outport
  Ty : Outport  Port=2
  wires:
  Va/1 -> Sum/1
  "Vb "/1 -> Gain/1
  Gain/1 -> Gain1/1, Sum/2
  Sum/1 -> Tx/1
  Gain1/1 -> Ty/1

== system foc5/Subsystem/SVPWM/Subsystem5/xyII ==
  Va : Inport
  "Vb " : Inport  Port=2
  Gain : Gain  Gain=1/sqrt(3)
  Gain1 : Gain  Gain=2
  Sum : Sum  Inputs=|+-
  Tx : Outport
  Ty : Outport  Port=2
  wires:
  Va/1 -> Sum/1
  "Vb "/1 -> Gain/1
  Gain/1 -> Gain1/1, Sum/2
  Gain1/1 -> Tx/1  "Ty'"
  Sum/1 -> Ty/1  "Tx'"

== system foc5/Subsystem/SVPWM/Subsystem5/xyIII ==
  Va : Inport
  "Vb " : Inport  Port=2
  Gain : Gain  Gain=1/sqrt(3)
  Gain1 : Gain  Gain=2
  Sum : Sum  Inputs=|+-
  Tx : Outport
  Ty : Outport  Port=2
  wires:
  Va/1 -> Sum/1
  "Vb "/1 -> Gain/1
  Gain/1 -> Gain1/1, Sum/2
  Sum/1 -> Tx/1  "Tx'"
  Gain1/1 -> Ty/1  "Ty'"

== system foc5/Subsystem/SVPWM/Subsystem5/xyIV ==
  Va : Inport
  "Vb " : Inport  Port=2
  Gain : Gain  Gain=1/sqrt(3)
  Gain1 : Gain  Gain=2
  Sum : Sum  Inputs=|+-
  Tx : Outport
  Ty : Outport  Port=2
  wires:
  Va/1 -> Sum/1
  "Vb "/1 -> Gain/1
  Gain/1 -> Gain1/1, Sum/2
  Sum/1 -> Ty/1  "Tx'"
  Gain1/1 -> Tx/1  "Ty'"

== system foc5/Subsystem/SVPWM/Subsystem5/xyV ==
  Va : Inport
  "Vb " : Inport  Port=2
  Gain : Gain  Gain=1/sqrt(3)
  Gain1 : Gain  Gain=2
  Sum : Sum  Inputs=|+-
  Tx : Outport
  Ty : Outport  Port=2
  wires:
  Va/1 -> Sum/1
  "Vb "/1 -> Gain/1
  Gain/1 -> Gain1/1, Sum/2
  Sum/1 -> Tx/1  "Tx'"
  Gain1/1 -> Ty/1  "Ty'"

== system foc5/Subsystem/SVPWM/Subsystem5/xyVI ==
  Va : Inport
  "Vb " : Inport  Port=2
  Gain : Gain  Gain=1/sqrt(3)
  Gain1 : Gain  Gain=2
  Sum : Sum  Inputs=|+-
  Tx : Outport
  Ty : Outport  Port=2
  wires:
  Va/1 -> Sum/1
  "Vb "/1 -> Gain/1
  Gain/1 -> Gain1/1, Sum/2
  Gain1/1 -> Tx/1  "Ty'"
  Sum/1 -> Ty/1  "Tx'"

== system foc5/Subsystem/SVPWM/Sec/Subsystem1/Subsystem ==
  Va : Inport
  "Vb " : Inport  Port=2
  Constant : Constant  Value=0
  Constant1 : Constant
  Gain : Gain  Gain=sqrt(3)
  Sum : Sum  Inputs=|-+
  Switch : Switch  Criteria=u2 > Threshold
  A : Outport
  wires:
  Va/1 -> Gain/1
  "Vb "/1 -> Sum/2
  Gain/1 -> Sum/1
  Switch/1 -> A/1
  Sum/1 -> Switch/2  "Vb-sqrt(3)*Va"
  Constant1/1 -> Switch/3
  Constant/1 -> Switch/1

== system foc5/Subsystem/SVPWM/Sec/Subsystem1/Subsystem1 ==
  Va : Inport
  "Vb " : Inport  Port=2
  Constant : Constant  Value=0
  Constant1 : Constant
  Gain : Gain  Gain=sqrt(3)
  Sum : Sum  Inputs=|++
  Switch : Switch  Criteria=u2 > Threshold
  B : Outport
  wires:
  Va/1 -> Gain/1
  "Vb "/1 -> Sum/2
  Gain/1 -> Sum/1
  Sum/1 -> Switch/2  "Vb+sqrt(3)*Va"
  Switch/1 -> B/1
  Constant/1 -> Switch/1
  Constant1/1 -> Switch/3

== system foc5/Subsystem/SVPWM/Sec/Subsystem1/Subsystem2 ==
  "Vb " : Inport
  Constant : Constant
  Constant1 : Constant  Value=-1
  Fcn : Fcn  Expr=0.5*u(1)+0.5
  Switch : Switch
  C : Outport
  wires:
  Fcn/1 -> C/1
  Switch/1 -> Fcn/1
  "Vb "/1 -> Switch/2
  Constant1/1 -> Switch/3
  Constant/1 -> Switch/1

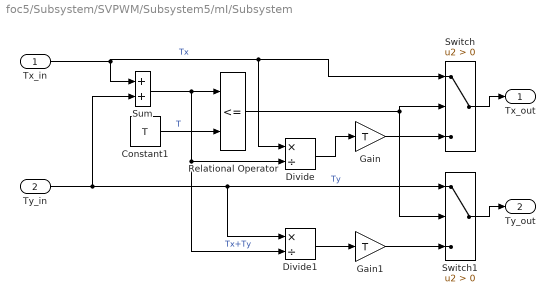
== system foc5/Subsystem/SVPWM/Subsystem5/mI/Subsystem ==
  Tx_in : Inport
  Ty_in : Inport  Port=2
  Constant1 : Constant  Value=T
  Divide : Product  Inputs=*/
  Divide1 : Product  Inputs=*/
  Gain : Gain  Gain=T
  Gain1 : Gain  Gain=T
  Relational Operator : RelationalOperator  Operator=<=  OutDataTypeStr=boolean  RndMeth=Simplest
  Sum : Sum
  Switch : Switch  Criteria=u2 > Threshold
  Switch1 : Switch  Criteria=u2 > Threshold
  Tx_out : Outport
  Ty_out : Outport  Port=2
  wires:
  Relational Operator/1 -> Switch1/2, Switch/2
  Tx_in/1 -> Divide/1, Switch/1, Sum/1  "Tx"
  Ty_in/1 -> Sum/2, Switch1/1, Divide1/1  "Ty"
  Sum/1 -> Divide1/2, Divide/2, Relational Operator/1  "Tx+Ty"
  Divide1/1 -> Gain1/1
  Constant1/1 -> Relational Operator/2  "T"
  Switch1/1 -> Ty_out/1
  Switch/1 -> Tx_out/1
  Divide/1 -> Gain/1
  Gain/1 -> Switch/3
  Gain1/1 -> Switch1/3

== system foc5/Subsystem/SVPWM/Subsystem5/mII/Subsystem ==
  Tx_in : Inport
  Ty_in : Inport  Port=2
  Constant1 : Constant  Value=T
  Divide : Product  Inputs=*/
  Divide1 : Product  Inputs=*/
  Gain : Gain  Gain=T
  Gain1 : Gain  Gain=T
  Relational Operator : RelationalOperator  Operator=<=  OutDataTypeStr=boolean  RndMeth=Simplest
  Sum : Sum
  Switch : Switch  Criteria=u2 > Threshold
  Switch1 : Switch  Criteria=u2 > Threshold
  Tx_out : Outport
  Ty_out : Outport  Port=2
  wires:
  Relational Operator/1 -> Switch1/2, Switch/2
  Tx_in/1 -> Divide/1, Switch/1, Sum/1  "T"
  Ty_in/1 -> Sum/2, Switch1/1, Divide1/1  "Ty"
  Sum/1 -> Divide1/2, Divide/2, Relational Operator/1  "Tx+Ty"
  Divide1/1 -> Gain1/1
  Constant1/1 -> Relational Operator/2  "T"
  Switch1/1 -> Ty_out/1
  Switch/1 -> Tx_out/1
  Divide/1 -> Gain/1
  Gain/1 -> Switch/3
  Gain1/1 -> Switch1/3

== system foc5/Subsystem/SVPWM/Subsystem5/mIII/Subsystem ==
  Tx_in : Inport
  Ty_in : Inport  Port=2
  Constant1 : Constant  Value=T
  Divide : Product  Inputs=*/
  Divide1 : Product  Inputs=*/
  Gain : Gain  Gain=T
  Gain1 : Gain  Gain=T
  Relational Operator : RelationalOperator  Operator=<=  OutDataTypeStr=boolean  RndMeth=Simplest
  Sum : Sum
  Switch : Switch  Criteria=u2 > Threshold
  Switch1 : Switch  Criteria=u2 > Threshold
  Tx_out : Outport
  Ty_out : Outport  Port=2
  wires:
  Relational Operator/1 -> Switch1/2, Switch/2
  Tx_in/1 -> Divide/1, Switch/1, Sum/1  "T"
  Ty_in/1 -> Sum/2, Switch1/1, Divide1/1  "Ty"
  Sum/1 -> Divide1/2, Divide/2, Relational Operator/1  "Tx+Ty"
  Divide1/1 -> Gain1/1
  Constant1/1 -> Relational Operator/2  "T"
  Switch1/1 -> Ty_out/1
  Switch/1 -> Tx_out/1
  Divide/1 -> Gain/1
  Gain/1 -> Switch/3
  Gain1/1 -> Switch1/3

== system foc5/Subsystem/SVPWM/Subsystem5/mIV/Subsystem ==
  Tx_in : Inport
  Ty_in : Inport  Port=2
  Constant1 : Constant  Value=T
  Divide : Product  Inputs=*/
  Divide1 : Product  Inputs=*/
  Gain : Gain  Gain=T
  Gain1 : Gain  Gain=T
  Relational Operator : RelationalOperator  Operator=<=  OutDataTypeStr=boolean  RndMeth=Simplest
  Sum : Sum
  Switch : Switch  Criteria=u2 > Threshold
  Switch1 : Switch  Criteria=u2 > Threshold
  Tx_out : Outport
  Ty_out : Outport  Port=2
  wires:
  Relational Operator/1 -> Switch1/2, Switch/2
  Tx_in/1 -> Divide/1, Switch/1, Sum/1  "T"
  Ty_in/1 -> Sum/2, Switch1/1, Divide1/1  "Ty"
  Sum/1 -> Divide1/2, Divide/2, Relational Operator/1  "Tx+Ty"
  Divide1/1 -> Gain1/1
  Constant1/1 -> Relational Operator/2  "T"
  Switch1/1 -> Ty_out/1
  Switch/1 -> Tx_out/1
  Divide/1 -> Gain/1
  Gain/1 -> Switch/3
  Gain1/1 -> Switch1/3

== system foc5/Subsystem/SVPWM/Subsystem5/mV/Subsystem ==
  Tx_in : Inport
  Ty_in : Inport  Port=2
  Constant1 : Constant  Value=T
  Divide : Product  Inputs=*/
  Divide1 : Product  Inputs=*/
  Gain : Gain  Gain=T
  Gain1 : Gain  Gain=T
  Relational Operator : RelationalOperator  Operator=<=  OutDataTypeStr=boolean  RndMeth=Simplest
  Sum : Sum
  Switch : Switch  Criteria=u2 > Threshold
  Switch1 : Switch  Criteria=u2 > Threshold
  Tx_out : Outport
  Ty_out : Outport  Port=2
  wires:
  Relational Operator/1 -> Switch1/2, Switch/2
  Tx_in/1 -> Divide/1, Switch/1, Sum/1  "T"
  Ty_in/1 -> Sum/2, Switch1/1, Divide1/1  "Ty"
  Sum/1 -> Divide1/2, Divide/2, Relational Operator/1  "Tx+Ty"
  Divide1/1 -> Gain1/1
  Constant1/1 -> Relational Operator/2  "T"
  Switch1/1 -> Ty_out/1
  Switch/1 -> Tx_out/1
  Divide/1 -> Gain/1
  Gain/1 -> Switch/3
  Gain1/1 -> Switch1/3

== system foc5/Subsystem/SVPWM/Subsystem5/mVI/Subsystem ==
  Tx_in : Inport
  Ty_in : Inport  Port=2
  Constant1 : Constant  Value=T
  Divide : Product  Inputs=*/
  Divide1 : Product  Inputs=*/
  Gain : Gain  Gain=T
  Gain1 : Gain  Gain=T
  Relational Operator : RelationalOperator  Operator=<=  OutDataTypeStr=boolean  RndMeth=Simplest
  Sum : Sum
  Switch : Switch  Criteria=u2 > Threshold
  Switch1 : Switch  Criteria=u2 > Threshold
  Tx_out : Outport
  Ty_out : Outport  Port=2
  wires:
  Relational Operator/1 -> Switch1/2, Switch/2
  Tx_in/1 -> Divide/1, Switch/1, Sum/1  "T"
  Ty_in/1 -> Sum/2, Switch1/1, Divide1/1  "Ty"
  Sum/1 -> Divide1/2, Divide/2, Relational Operator/1  "Tx+Ty"
  Divide1/1 -> Gain1/1
  Constant1/1 -> Relational Operator/2  "T"
  Switch1/1 -> Ty_out/1
  Switch/1 -> Tx_out/1
  Divide/1 -> Gain/1
  Gain/1 -> Switch/3
  Gain1/1 -> Switch1/3
